simulink model "adsl_sim"  (Simulink 6.0)
settings: Solver=ode45  SolverMode=SingleTasking  StartTime=0.0  StopTime=2  RelTol=1e-3
PreLoadFcn:
  | % variables are initialized through the Model Workspace
model workspace: external: M-Code (data not in the file)
values from neighbouring files (symbols this model uses):
  H = conv2(chCoeff',W)    [eq_computecostfcn.m]    (also in eq_costfcnconverg.m = conv2(eq.chCoeff,W))
undefined symbols (not defined in the file or in its folder): b, rsgenpoly, slcm
libraries: commdigbbndam2 x512, simulink x37, commutil2 x8, commblkcod2 x4, commsequence2 x4, commsink2 x4, commcrc2 x4, commcnvintrlv2 x2, dspxfrm3 x2, dspsrcs4 x2, dspsigattribs x1, dspmtrx3 x1
(part 4 of 5)

== system adsl_sim/DMT Modulator/Modulator Bank 11 ==
  In1 : Inport  LatchInput=off
  Demux1 : Demux  Outputs=b(offset+1:offset+16)
  Matrix Concatenation : simulink/Math Operations/Matrix Concatenation  numInports=16  catMethod=Vertical
  Rectangular QAM Modulator Baseband1 : commdigbbndam2/Rectangular QAM Modulator Baseband  M=2^b(offset+1)  InType=Bit  Enc=Gray  PowType=Average Power  MinDist=2  AvgPow=1  PeakPow=1  Ph=0  numSamp=1
  Rectangular QAM Modulator Baseband10 : commdigbbndam2/Rectangular QAM Modulator Baseband  M=2^b(offset+10)  InType=Bit  Enc=Gray  PowType=Average Power  MinDist=2  AvgPow=1  PeakPow=1  Ph=0  numSamp=1
  Rectangular QAM Modulator Baseband11 : commdigbbndam2/Rectangular QAM Modulator Baseband  M=2^b(offset+11)  InType=Bit  Enc=Gray  PowType=Average Power  MinDist=2  AvgPow=1  PeakPow=1  Ph=0  numSamp=1
  Rectangular QAM Modulator Baseband12 : commdigbbndam2/Rectangular QAM Modulator Baseband  M=2^b(offset+12)  InType=Bit  Enc=Gray  PowType=Average Power  MinDist=2  AvgPow=1  PeakPow=1  Ph=0  numSamp=1
  Rectangular QAM Modulator Baseband13 : commdigbbndam2/Rectangular QAM Modulator Baseband  M=2^b(offset+13)  InType=Bit  Enc=Gray  PowType=Average Power  MinDist=2  AvgPow=1  PeakPow=1  Ph=0  numSamp=1
  Rectangular QAM Modulator Baseband14 : commdigbbndam2/Rectangular QAM Modulator Baseband  M=2^b(offset+14)  InType=Bit  Enc=Gray  PowType=Average Power  MinDist=2  AvgPow=1  PeakPow=1  Ph=0  numSamp=1
  Rectangular QAM Modulator Baseband15 : commdigbbndam2/Rectangular QAM Modulator Baseband  M=2^b(offset+15)  InType=Bit  Enc=Gray  PowType=Average Power  MinDist=2  AvgPow=1  PeakPow=1  Ph=0  numSamp=1
  Rectangular QAM Modulator Baseband16 : commdigbbndam2/Rectangular QAM Modulator Baseband  M=2^b(offset+16)  InType=Bit  Enc=Gray  PowType=Average Power  MinDist=2  AvgPow=1  PeakPow=1  Ph=0  numSamp=1
  Rectangular QAM Modulator Baseband2 : commdigbbndam2/Rectangular QAM Modulator Baseband  M=2^b(offset+2)  InType=Bit  Enc=Gray  PowType=Average Power  MinDist=2  AvgPow=1  PeakPow=1  Ph=0  numSamp=1
  Rectangular QAM Modulator Baseband3 : commdigbbndam2/Rectangular QAM Modulator Baseband  M=2^b(offset+3)  InType=Bit  Enc=Gray  PowType=Average Power  MinDist=2  AvgPow=1  PeakPow=1  Ph=0  numSamp=1
  Rectangular QAM Modulator Baseband4 : commdigbbndam2/Rectangular QAM Modulator Baseband  M=2^b(offset+4)  InType=Bit  Enc=Gray  PowType=Average Power  MinDist=2  AvgPow=1  PeakPow=1  Ph=0  numSamp=1
  Rectangular QAM Modulator Baseband5 : commdigbbndam2/Rectangular QAM Modulator Baseband  M=2^b(offset+5)  InType=Bit  Enc=Gray  PowType=Average Power  MinDist=2  AvgPow=1  PeakPow=1  Ph=0  numSamp=1
  Rectangular QAM Modulator Baseband6 : commdigbbndam2/Rectangular QAM Modulator Baseband  M=2^b(offset+6)  InType=Bit  Enc=Gray  PowType=Average Power  MinDist=2  AvgPow=1  PeakPow=1  Ph=0  numSamp=1
  Rectangular QAM Modulator Baseband7 : commdigbbndam2/Rectangular QAM Modulator Baseband  M=2^b(offset+7)  InType=Bit  Enc=Gray  PowType=Average Power  MinDist=2  AvgPow=1  PeakPow=1  Ph=0  numSamp=1
  Rectangular QAM Modulator Baseband8 : commdigbbndam2/Rectangular QAM Modulator Baseband  M=2^b(offset+8)  InType=Bit  Enc=Gray  PowType=Average Power  MinDist=2  AvgPow=1  PeakPow=1  Ph=0  numSamp=1
  Rectangular QAM Modulator Baseband9 : commdigbbndam2/Rectangular QAM Modulator Baseband  M=2^b(offset+9)  InType=Bit  Enc=Gray  PowType=Average Power  MinDist=2  AvgPow=1  PeakPow=1  Ph=0  numSamp=1
  Out1 : Outport
  wires:
  Rectangular QAM Modulator Baseband16/1 -> Matrix Concatenation/16
  Rectangular QAM Modulator Baseband15/1 -> Matrix Concatenation/15
  Rectangular QAM Modulator Baseband14/1 -> Matrix Concatenation/14
  Rectangular QAM Modulator Baseband13/1 -> Matrix Concatenation/13
  Rectangular QAM Modulator Baseband12/1 -> Matrix Concatenation/12
  Rectangular QAM Modulator Baseband11/1 -> Matrix Concatenation/11
  Rectangular QAM Modulator Baseband10/1 -> Matrix Concatenation/10
  Rectangular QAM Modulator Baseband9/1 -> Matrix Concatenation/9
  Rectangular QAM Modulator Baseband8/1 -> Matrix Concatenation/8
  Rectangular QAM Modulator Baseband7/1 -> Matrix Concatenation/7
  Rectangular QAM Modulator Baseband6/1 -> Matrix Concatenation/6
  Rectangular QAM Modulator Baseband5/1 -> Matrix Concatenation/5
  Rectangular QAM Modulator Baseband4/1 -> Matrix Concatenation/4
  Rectangular QAM Modulator Baseband3/1 -> Matrix Concatenation/3
  Rectangular QAM Modulator Baseband2/1 -> Matrix Concatenation/2
  Demux1/16 -> Rectangular QAM Modulator Baseband16/1
  Demux1/15 -> Rectangular QAM Modulator Baseband15/1
  Demux1/14 -> Rectangular QAM Modulator Baseband14/1
  Demux1/13 -> Rectangular QAM Modulator Baseband13/1
  Demux1/12 -> Rectangular QAM Modulator Baseband12/1
  Demux1/11 -> Rectangular QAM Modulator Baseband11/1
  Demux1/10 -> Rectangular QAM Modulator Baseband10/1
  Demux1/9 -> Rectangular QAM Modulator Baseband9/1
  Demux1/8 -> Rectangular QAM Modulator Baseband8/1
  Demux1/7 -> Rectangular QAM Modulator Baseband7/1
  Demux1/6 -> Rectangular QAM Modulator Baseband6/1
  Demux1/5 -> Rectangular QAM Modulator Baseband5/1
  Demux1/4 -> Rectangular QAM Modulator Baseband4/1
  Demux1/3 -> Rectangular QAM Modulator Baseband3/1
  Matrix Concatenation/1 -> Out1/1
  In1/1 -> Demux1/1
  Demux1/2 -> Rectangular QAM Modulator Baseband2/1
  Demux1/1 -> Rectangular QAM Modulator Baseband1/1
  Rectangular QAM Modulator Baseband1/1 -> Matrix Concatenation/1

== system adsl_sim/DMT Modulator/Modulator Bank 12 ==
  In1 : Inport  LatchInput=off
  Demux1 : Demux  Outputs=b(offset+1:offset+16)
  Matrix Concatenation : simulink/Math Operations/Matrix Concatenation  numInports=16  catMethod=Vertical
  Rectangular QAM Modulator Baseband1 : commdigbbndam2/Rectangular QAM Modulator Baseband  M=2^b(offset+1)  InType=Bit  Enc=Gray  PowType=Average Power  MinDist=2  AvgPow=1  PeakPow=1  Ph=0  numSamp=1
  Rectangular QAM Modulator Baseband10 : commdigbbndam2/Rectangular QAM Modulator Baseband  M=2^b(offset+10)  InType=Bit  Enc=Gray  PowType=Average Power  MinDist=2  AvgPow=1  PeakPow=1  Ph=0  numSamp=1
  Rectangular QAM Modulator Baseband11 : commdigbbndam2/Rectangular QAM Modulator Baseband  M=2^b(offset+11)  InType=Bit  Enc=Gray  PowType=Average Power  MinDist=2  AvgPow=1  PeakPow=1  Ph=0  numSamp=1
  Rectangular QAM Modulator Baseband12 : commdigbbndam2/Rectangular QAM Modulator Baseband  M=2^b(offset+12)  InType=Bit  Enc=Gray  PowType=Average Power  MinDist=2  AvgPow=1  PeakPow=1  Ph=0  numSamp=1
  Rectangular QAM Modulator Baseband13 : commdigbbndam2/Rectangular QAM Modulator Baseband  M=2^b(offset+13)  InType=Bit  Enc=Gray  PowType=Average Power  MinDist=2  AvgPow=1  PeakPow=1  Ph=0  numSamp=1
  Rectangular QAM Modulator Baseband14 : commdigbbndam2/Rectangular QAM Modulator Baseband  M=2^b(offset+14)  InType=Bit  Enc=Gray  PowType=Average Power  MinDist=2  AvgPow=1  PeakPow=1  Ph=0  numSamp=1
  Rectangular QAM Modulator Baseband15 : commdigbbndam2/Rectangular QAM Modulator Baseband  M=2^b(offset+15)  InType=Bit  Enc=Gray  PowType=Average Power  MinDist=2  AvgPow=1  PeakPow=1  Ph=0  numSamp=1
  Rectangular QAM Modulator Baseband16 : commdigbbndam2/Rectangular QAM Modulator Baseband  M=2^b(offset+16)  InType=Bit  Enc=Gray  PowType=Average Power  MinDist=2  AvgPow=1  PeakPow=1  Ph=0  numSamp=1
  Rectangular QAM Modulator Baseband2 : commdigbbndam2/Rectangular QAM Modulator Baseband  M=2^b(offset+2)  InType=Bit  Enc=Gray  PowType=Average Power  MinDist=2  AvgPow=1  PeakPow=1  Ph=0  numSamp=1
  Rectangular QAM Modulator Baseband3 : commdigbbndam2/Rectangular QAM Modulator Baseband  M=2^b(offset+3)  InType=Bit  Enc=Gray  PowType=Average Power  MinDist=2  AvgPow=1  PeakPow=1  Ph=0  numSamp=1
  Rectangular QAM Modulator Baseband4 : commdigbbndam2/Rectangular QAM Modulator Baseband  M=2^b(offset+4)  InType=Bit  Enc=Gray  PowType=Average Power  MinDist=2  AvgPow=1  PeakPow=1  Ph=0  numSamp=1
  Rectangular QAM Modulator Baseband5 : commdigbbndam2/Rectangular QAM Modulator Baseband  M=2^b(offset+5)  InType=Bit  Enc=Gray  PowType=Average Power  MinDist=2  AvgPow=1  PeakPow=1  Ph=0  numSamp=1
  Rectangular QAM Modulator Baseband6 : commdigbbndam2/Rectangular QAM Modulator Baseband  M=2^b(offset+6)  InType=Bit  Enc=Gray  PowType=Average Power  MinDist=2  AvgPow=1  PeakPow=1  Ph=0  numSamp=1
  Rectangular QAM Modulator Baseband7 : commdigbbndam2/Rectangular QAM Modulator Baseband  M=2^b(offset+7)  InType=Bit  Enc=Gray  PowType=Average Power  MinDist=2  AvgPow=1  PeakPow=1  Ph=0  numSamp=1
  Rectangular QAM Modulator Baseband8 : commdigbbndam2/Rectangular QAM Modulator Baseband  M=2^b(offset+8)  InType=Bit  Enc=Gray  PowType=Average Power  MinDist=2  AvgPow=1  PeakPow=1  Ph=0  numSamp=1
  Rectangular QAM Modulator Baseband9 : commdigbbndam2/Rectangular QAM Modulator Baseband  M=2^b(offset+9)  InType=Bit  Enc=Gray  PowType=Average Power  MinDist=2  AvgPow=1  PeakPow=1  Ph=0  numSamp=1
  Out1 : Outport
  wires:
  Rectangular QAM Modulator Baseband1/1 -> Matrix Concatenation/1
  Demux1/1 -> Rectangular QAM Modulator Baseband1/1
  Demux1/2 -> Rectangular QAM Modulator Baseband2/1
  In1/1 -> Demux1/1
  Matrix Concatenation/1 -> Out1/1
  Demux1/3 -> Rectangular QAM Modulator Baseband3/1
  Demux1/4 -> Rectangular QAM Modulator Baseband4/1
  Demux1/5 -> Rectangular QAM Modulator Baseband5/1
  Demux1/6 -> Rectangular QAM Modulator Baseband6/1
  Demux1/7 -> Rectangular QAM Modulator Baseband7/1
  Demux1/8 -> Rectangular QAM Modulator Baseband8/1
  Demux1/9 -> Rectangular QAM Modulator Baseband9/1
  Demux1/10 -> Rectangular QAM Modulator Baseband10/1
  Demux1/11 -> Rectangular QAM Modulator Baseband11/1
  Demux1/12 -> Rectangular QAM Modulator Baseband12/1
  Demux1/13 -> Rectangular QAM Modulator Baseband13/1
  Demux1/14 -> Rectangular QAM Modulator Baseband14/1
  Demux1/15 -> Rectangular QAM Modulator Baseband15/1
  Demux1/16 -> Rectangular QAM Modulator Baseband16/1
  Rectangular QAM Modulator Baseband2/1 -> Matrix Concatenation/2
  Rectangular QAM Modulator Baseband3/1 -> Matrix Concatenation/3
  Rectangular QAM Modulator Baseband4/1 -> Matrix Concatenation/4
  Rectangular QAM Modulator Baseband5/1 -> Matrix Concatenation/5
  Rectangular QAM Modulator Baseband6/1 -> Matrix Concatenation/6
  Rectangular QAM Modulator Baseband7/1 -> Matrix Concatenation/7
  Rectangular QAM Modulator Baseband8/1 -> Matrix Concatenation/8
  Rectangular QAM Modulator Baseband9/1 -> Matrix Concatenation/9
  Rectangular QAM Modulator Baseband10/1 -> Matrix Concatenation/10
  Rectangular QAM Modulator Baseband11/1 -> Matrix Concatenation/11
  Rectangular QAM Modulator Baseband12/1 -> Matrix Concatenation/12
  Rectangular QAM Modulator Baseband13/1 -> Matrix Concatenation/13
  Rectangular QAM Modulator Baseband14/1 -> Matrix Concatenation/14
  Rectangular QAM Modulator Baseband15/1 -> Matrix Concatenation/15
  Rectangular QAM Modulator Baseband16/1 -> Matrix Concatenation/16

== system adsl_sim/DMT Modulator/Modulator Bank 13 ==
  In1 : Inport  LatchInput=off
  Demux1 : Demux  Outputs=b(offset+1:offset+16)
  Matrix Concatenation : simulink/Math Operations/Matrix Concatenation  numInports=16  catMethod=Vertical
  Rectangular QAM Modulator Baseband1 : commdigbbndam2/Rectangular QAM Modulator Baseband  M=2^b(offset+1)  InType=Bit  Enc=Gray  PowType=Average Power  MinDist=2  AvgPow=1  PeakPow=1  Ph=0  numSamp=1
  Rectangular QAM Modulator Baseband10 : commdigbbndam2/Rectangular QAM Modulator Baseband  M=2^b(offset+10)  InType=Bit  Enc=Gray  PowType=Average Power  MinDist=2  AvgPow=1  PeakPow=1  Ph=0  numSamp=1
  Rectangular QAM Modulator Baseband11 : commdigbbndam2/Rectangular QAM Modulator Baseband  M=2^b(offset+11)  InType=Bit  Enc=Gray  PowType=Average Power  MinDist=2  AvgPow=1  PeakPow=1  Ph=0  numSamp=1
  Rectangular QAM Modulator Baseband12 : commdigbbndam2/Rectangular QAM Modulator Baseband  M=2^b(offset+12)  InType=Bit  Enc=Gray  PowType=Average Power  MinDist=2  AvgPow=1  PeakPow=1  Ph=0  numSamp=1
  Rectangular QAM Modulator Baseband13 : commdigbbndam2/Rectangular QAM Modulator Baseband  M=2^b(offset+13)  InType=Bit  Enc=Gray  PowType=Average Power  MinDist=2  AvgPow=1  PeakPow=1  Ph=0  numSamp=1
  Rectangular QAM Modulator Baseband14 : commdigbbndam2/Rectangular QAM Modulator Baseband  M=2^b(offset+14)  InType=Bit  Enc=Gray  PowType=Average Power  MinDist=2  AvgPow=1  PeakPow=1  Ph=0  numSamp=1
  Rectangular QAM Modulator Baseband15 : commdigbbndam2/Rectangular QAM Modulator Baseband  M=2^b(offset+15)  InType=Bit  Enc=Gray  PowType=Average Power  MinDist=2  AvgPow=1  PeakPow=1  Ph=0  numSamp=1
  Rectangular QAM Modulator Baseband16 : commdigbbndam2/Rectangular QAM Modulator Baseband  M=2^b(offset+16)  InType=Bit  Enc=Gray  PowType=Average Power  MinDist=2  AvgPow=1  PeakPow=1  Ph=0  numSamp=1
  Rectangular QAM Modulator Baseband2 : commdigbbndam2/Rectangular QAM Modulator Baseband  M=2^b(offset+2)  InType=Bit  Enc=Gray  PowType=Average Power  MinDist=2  AvgPow=1  PeakPow=1  Ph=0  numSamp=1
  Rectangular QAM Modulator Baseband3 : commdigbbndam2/Rectangular QAM Modulator Baseband  M=2^b(offset+3)  InType=Bit  Enc=Gray  PowType=Average Power  MinDist=2  AvgPow=1  PeakPow=1  Ph=0  numSamp=1
  Rectangular QAM Modulator Baseband4 : commdigbbndam2/Rectangular QAM Modulator Baseband  M=2^b(offset+4)  InType=Bit  Enc=Gray  PowType=Average Power  MinDist=2  AvgPow=1  PeakPow=1  Ph=0  numSamp=1
  Rectangular QAM Modulator Baseband5 : commdigbbndam2/Rectangular QAM Modulator Baseband  M=2^b(offset+5)  InType=Bit  Enc=Gray  PowType=Average Power  MinDist=2  AvgPow=1  PeakPow=1  Ph=0  numSamp=1
  Rectangular QAM Modulator Baseband6 : commdigbbndam2/Rectangular QAM Modulator Baseband  M=2^b(offset+6)  InType=Bit  Enc=Gray  PowType=Average Power  MinDist=2  AvgPow=1  PeakPow=1  Ph=0  numSamp=1
  Rectangular QAM Modulator Baseband7 : commdigbbndam2/Rectangular QAM Modulator Baseband  M=2^b(offset+7)  InType=Bit  Enc=Gray  PowType=Average Power  MinDist=2  AvgPow=1  PeakPow=1  Ph=0  numSamp=1
  Rectangular QAM Modulator Baseband8 : commdigbbndam2/Rectangular QAM Modulator Baseband  M=2^b(offset+8)  InType=Bit  Enc=Gray  PowType=Average Power  MinDist=2  AvgPow=1  PeakPow=1  Ph=0  numSamp=1
  Rectangular QAM Modulator Baseband9 : commdigbbndam2/Rectangular QAM Modulator Baseband  M=2^b(offset+9)  InType=Bit  Enc=Gray  PowType=Average Power  MinDist=2  AvgPow=1  PeakPow=1  Ph=0  numSamp=1
  Out1 : Outport
  wires:
  Rectangular QAM Modulator Baseband16/1 -> Matrix Concatenation/16
  Rectangular QAM Modulator Baseband15/1 -> Matrix Concatenation/15
  Rectangular QAM Modulator Baseband14/1 -> Matrix Concatenation/14
  Rectangular QAM Modulator Baseband13/1 -> Matrix Concatenation/13
  Rectangular QAM Modulator Baseband12/1 -> Matrix Concatenation/12
  Rectangular QAM Modulator Baseband11/1 -> Matrix Concatenation/11
  Rectangular QAM Modulator Baseband10/1 -> Matrix Concatenation/10
  Rectangular QAM Modulator Baseband9/1 -> Matrix Concatenation/9
  Rectangular QAM Modulator Baseband8/1 -> Matrix Concatenation/8
  Rectangular QAM Modulator Baseband7/1 -> Matrix Concatenation/7
  Rectangular QAM Modulator Baseband6/1 -> Matrix Concatenation/6
  Rectangular QAM Modulator Baseband5/1 -> Matrix Concatenation/5
  Rectangular QAM Modulator Baseband4/1 -> Matrix Concatenation/4
  Rectangular QAM Modulator Baseband3/1 -> Matrix Concatenation/3
  Rectangular QAM Modulator Baseband2/1 -> Matrix Concatenation/2
  Demux1/16 -> Rectangular QAM Modulator Baseband16/1
  Demux1/15 -> Rectangular QAM Modulator Baseband15/1
  Demux1/14 -> Rectangular QAM Modulator Baseband14/1
  Demux1/13 -> Rectangular QAM Modulator Baseband13/1
  Demux1/12 -> Rectangular QAM Modulator Baseband12/1
  Demux1/11 -> Rectangular QAM Modulator Baseband11/1
  Demux1/10 -> Rectangular QAM Modulator Baseband10/1
  Demux1/9 -> Rectangular QAM Modulator Baseband9/1
  Demux1/8 -> Rectangular QAM Modulator Baseband8/1
  Demux1/7 -> Rectangular QAM Modulator Baseband7/1
  Demux1/6 -> Rectangular QAM Modulator Baseband6/1
  Demux1/5 -> Rectangular QAM Modulator Baseband5/1
  Demux1/4 -> Rectangular QAM Modulator Baseband4/1
  Demux1/3 -> Rectangular QAM Modulator Baseband3/1
  Matrix Concatenation/1 -> Out1/1
  In1/1 -> Demux1/1
  Demux1/2 -> Rectangular QAM Modulator Baseband2/1
  Demux1/1 -> Rectangular QAM Modulator Baseband1/1
  Rectangular QAM Modulator Baseband1/1 -> Matrix Concatenation/1

== system adsl_sim/DMT Modulator/Modulator Bank 14 ==
  In1 : Inport  LatchInput=off
  Demux1 : Demux  Outputs=b(offset+1:offset+16)
  Matrix Concatenation : simulink/Math Operations/Matrix Concatenation  numInports=16  catMethod=Vertical
  Rectangular QAM Modulator Baseband1 : commdigbbndam2/Rectangular QAM Modulator Baseband  M=2^b(offset+1)  InType=Bit  Enc=Gray  PowType=Average Power  MinDist=2  AvgPow=1  PeakPow=1  Ph=0  numSamp=1
  Rectangular QAM Modulator Baseband10 : commdigbbndam2/Rectangular QAM Modulator Baseband  M=2^b(offset+10)  InType=Bit  Enc=Gray  PowType=Average Power  MinDist=2  AvgPow=1  PeakPow=1  Ph=0  numSamp=1
  Rectangular QAM Modulator Baseband11 : commdigbbndam2/Rectangular QAM Modulator Baseband  M=2^b(offset+11)  InType=Bit  Enc=Gray  PowType=Average Power  MinDist=2  AvgPow=1  PeakPow=1  Ph=0  numSamp=1
  Rectangular QAM Modulator Baseband12 : commdigbbndam2/Rectangular QAM Modulator Baseband  M=2^b(offset+12)  InType=Bit  Enc=Gray  PowType=Average Power  MinDist=2  AvgPow=1  PeakPow=1  Ph=0  numSamp=1
  Rectangular QAM Modulator Baseband13 : commdigbbndam2/Rectangular QAM Modulator Baseband  M=2^b(offset+13)  InType=Bit  Enc=Gray  PowType=Average Power  MinDist=2  AvgPow=1  PeakPow=1  Ph=0  numSamp=1
  Rectangular QAM Modulator Baseband14 : commdigbbndam2/Rectangular QAM Modulator Baseband  M=2^b(offset+14)  InType=Bit  Enc=Gray  PowType=Average Power  MinDist=2  AvgPow=1  PeakPow=1  Ph=0  numSamp=1
  Rectangular QAM Modulator Baseband15 : commdigbbndam2/Rectangular QAM Modulator Baseband  M=2^b(offset+15)  InType=Bit  Enc=Gray  PowType=Average Power  MinDist=2  AvgPow=1  PeakPow=1  Ph=0  numSamp=1
  Rectangular QAM Modulator Baseband16 : commdigbbndam2/Rectangular QAM Modulator Baseband  M=2^b(offset+16)  InType=Bit  Enc=Gray  PowType=Average Power  MinDist=2  AvgPow=1  PeakPow=1  Ph=0  numSamp=1
  Rectangular QAM Modulator Baseband2 : commdigbbndam2/Rectangular QAM Modulator Baseband  M=2^b(offset+2)  InType=Bit  Enc=Gray  PowType=Average Power  MinDist=2  AvgPow=1  PeakPow=1  Ph=0  numSamp=1
  Rectangular QAM Modulator Baseband3 : commdigbbndam2/Rectangular QAM Modulator Baseband  M=2^b(offset+3)  InType=Bit  Enc=Gray  PowType=Average Power  MinDist=2  AvgPow=1  PeakPow=1  Ph=0  numSamp=1
  Rectangular QAM Modulator Baseband4 : commdigbbndam2/Rectangular QAM Modulator Baseband  M=2^b(offset+4)  InType=Bit  Enc=Gray  PowType=Average Power  MinDist=2  AvgPow=1  PeakPow=1  Ph=0  numSamp=1
  Rectangular QAM Modulator Baseband5 : commdigbbndam2/Rectangular QAM Modulator Baseband  M=2^b(offset+5)  InType=Bit  Enc=Gray  PowType=Average Power  MinDist=2  AvgPow=1  PeakPow=1  Ph=0  numSamp=1
  Rectangular QAM Modulator Baseband6 : commdigbbndam2/Rectangular QAM Modulator Baseband  M=2^b(offset+6)  InType=Bit  Enc=Gray  PowType=Average Power  MinDist=2  AvgPow=1  PeakPow=1  Ph=0  numSamp=1
  Rectangular QAM Modulator Baseband7 : commdigbbndam2/Rectangular QAM Modulator Baseband  M=2^b(offset+7)  InType=Bit  Enc=Gray  PowType=Average Power  MinDist=2  AvgPow=1  PeakPow=1  Ph=0  numSamp=1
  Rectangular QAM Modulator Baseband8 : commdigbbndam2/Rectangular QAM Modulator Baseband  M=2^b(offset+8)  InType=Bit  Enc=Gray  PowType=Average Power  MinDist=2  AvgPow=1  PeakPow=1  Ph=0  numSamp=1
  Rectangular QAM Modulator Baseband9 : commdigbbndam2/Rectangular QAM Modulator Baseband  M=2^b(offset+9)  InType=Bit  Enc=Gray  PowType=Average Power  MinDist=2  AvgPow=1  PeakPow=1  Ph=0  numSamp=1
  Out1 : Outport
  wires:
  Rectangular QAM Modulator Baseband1/1 -> Matrix Concatenation/1
  Demux1/1 -> Rectangular QAM Modulator Baseband1/1
  Demux1/2 -> Rectangular QAM Modulator Baseband2/1
  In1/1 -> Demux1/1
  Matrix Concatenation/1 -> Out1/1
  Demux1/3 -> Rectangular QAM Modulator Baseband3/1
  Demux1/4 -> Rectangular QAM Modulator Baseband4/1
  Demux1/5 -> Rectangular QAM Modulator Baseband5/1
  Demux1/6 -> Rectangular QAM Modulator Baseband6/1
  Demux1/7 -> Rectangular QAM Modulator Baseband7/1
  Demux1/8 -> Rectangular QAM Modulator Baseband8/1
  Demux1/9 -> Rectangular QAM Modulator Baseband9/1
  Demux1/10 -> Rectangular QAM Modulator Baseband10/1
  Demux1/11 -> Rectangular QAM Modulator Baseband11/1
  Demux1/12 -> Rectangular QAM Modulator Baseband12/1
  Demux1/13 -> Rectangular QAM Modulator Baseband13/1
  Demux1/14 -> Rectangular QAM Modulator Baseband14/1
  Demux1/15 -> Rectangular QAM Modulator Baseband15/1
  Demux1/16 -> Rectangular QAM Modulator Baseband16/1
  Rectangular QAM Modulator Baseband2/1 -> Matrix Concatenation/2
  Rectangular QAM Modulator Baseband3/1 -> Matrix Concatenation/3
  Rectangular QAM Modulator Baseband4/1 -> Matrix Concatenation/4
  Rectangular QAM Modulator Baseband5/1 -> Matrix Concatenation/5
  Rectangular QAM Modulator Baseband6/1 -> Matrix Concatenation/6
  Rectangular QAM Modulator Baseband7/1 -> Matrix Concatenation/7
  Rectangular QAM Modulator Baseband8/1 -> Matrix Concatenation/8
  Rectangular QAM Modulator Baseband9/1 -> Matrix Concatenation/9
  Rectangular QAM Modulator Baseband10/1 -> Matrix Concatenation/10
  Rectangular QAM Modulator Baseband11/1 -> Matrix Concatenation/11
  Rectangular QAM Modulator Baseband12/1 -> Matrix Concatenation/12
  Rectangular QAM Modulator Baseband13/1 -> Matrix Concatenation/13
  Rectangular QAM Modulator Baseband14/1 -> Matrix Concatenation/14
  Rectangular QAM Modulator Baseband15/1 -> Matrix Concatenation/15
  Rectangular QAM Modulator Baseband16/1 -> Matrix Concatenation/16

== system adsl_sim/DMT Modulator/Modulator Bank 15 ==
  In1 : Inport  LatchInput=off
  Demux1 : Demux  Outputs=b(offset+1:offset+16)
  Matrix Concatenation : simulink/Math Operations/Matrix Concatenation  numInports=16  catMethod=Vertical
  Rectangular QAM Modulator Baseband1 : commdigbbndam2/Rectangular QAM Modulator Baseband  M=2^b(offset+1)  InType=Bit  Enc=Gray  PowType=Average Power  MinDist=2  AvgPow=1  PeakPow=1  Ph=0  numSamp=1
  Rectangular QAM Modulator Baseband10 : commdigbbndam2/Rectangular QAM Modulator Baseband  M=2^b(offset+10)  InType=Bit  Enc=Gray  PowType=Average Power  MinDist=2  AvgPow=1  PeakPow=1  Ph=0  numSamp=1
  Rectangular QAM Modulator Baseband11 : commdigbbndam2/Rectangular QAM Modulator Baseband  M=2^b(offset+11)  InType=Bit  Enc=Gray  PowType=Average Power  MinDist=2  AvgPow=1  PeakPow=1  Ph=0  numSamp=1
  Rectangular QAM Modulator Baseband12 : commdigbbndam2/Rectangular QAM Modulator Baseband  M=2^b(offset+12)  InType=Bit  Enc=Gray  PowType=Average Power  MinDist=2  AvgPow=1  PeakPow=1  Ph=0  numSamp=1
  Rectangular QAM Modulator Baseband13 : commdigbbndam2/Rectangular QAM Modulator Baseband  M=2^b(offset+13)  InType=Bit  Enc=Gray  PowType=Average Power  MinDist=2  AvgPow=1  PeakPow=1  Ph=0  numSamp=1
  Rectangular QAM Modulator Baseband14 : commdigbbndam2/Rectangular QAM Modulator Baseband  M=2^b(offset+14)  InType=Bit  Enc=Gray  PowType=Average Power  MinDist=2  AvgPow=1  PeakPow=1  Ph=0  numSamp=1
  Rectangular QAM Modulator Baseband15 : commdigbbndam2/Rectangular QAM Modulator Baseband  M=2^b(offset+15)  InType=Bit  Enc=Gray  PowType=Average Power  MinDist=2  AvgPow=1  PeakPow=1  Ph=0  numSamp=1
  Rectangular QAM Modulator Baseband16 : commdigbbndam2/Rectangular QAM Modulator Baseband  M=2^b(offset+16)  InType=Bit  Enc=Gray  PowType=Average Power  MinDist=2  AvgPow=1  PeakPow=1  Ph=0  numSamp=1
  Rectangular QAM Modulator Baseband2 : commdigbbndam2/Rectangular QAM Modulator Baseband  M=2^b(offset+2)  InType=Bit  Enc=Gray  PowType=Average Power  MinDist=2  AvgPow=1  PeakPow=1  Ph=0  numSamp=1
  Rectangular QAM Modulator Baseband3 : commdigbbndam2/Rectangular QAM Modulator Baseband  M=2^b(offset+3)  InType=Bit  Enc=Gray  PowType=Average Power  MinDist=2  AvgPow=1  PeakPow=1  Ph=0  numSamp=1
  Rectangular QAM Modulator Baseband4 : commdigbbndam2/Rectangular QAM Modulator Baseband  M=2^b(offset+4)  InType=Bit  Enc=Gray  PowType=Average Power  MinDist=2  AvgPow=1  PeakPow=1  Ph=0  numSamp=1
  Rectangular QAM Modulator Baseband5 : commdigbbndam2/Rectangular QAM Modulator Baseband  M=2^b(offset+5)  InType=Bit  Enc=Gray  PowType=Average Power  MinDist=2  AvgPow=1  PeakPow=1  Ph=0  numSamp=1
  Rectangular QAM Modulator Baseband6 : commdigbbndam2/Rectangular QAM Modulator Baseband  M=2^b(offset+6)  InType=Bit  Enc=Gray  PowType=Average Power  MinDist=2  AvgPow=1  PeakPow=1  Ph=0  numSamp=1
  Rectangular QAM Modulator Baseband7 : commdigbbndam2/Rectangular QAM Modulator Baseband  M=2^b(offset+7)  InType=Bit  Enc=Gray  PowType=Average Power  MinDist=2  AvgPow=1  PeakPow=1  Ph=0  numSamp=1
  Rectangular QAM Modulator Baseband8 : commdigbbndam2/Rectangular QAM Modulator Baseband  M=2^b(offset+8)  InType=Bit  Enc=Gray  PowType=Average Power  MinDist=2  AvgPow=1  PeakPow=1  Ph=0  numSamp=1
  Rectangular QAM Modulator Baseband9 : commdigbbndam2/Rectangular QAM Modulator Baseband  M=2^b(offset+9)  InType=Bit  Enc=Gray  PowType=Average Power  MinDist=2  AvgPow=1  PeakPow=1  Ph=0  numSamp=1
  Out1 : Outport
  wires:
  Rectangular QAM Modulator Baseband16/1 -> Matrix Concatenation/16
  Rectangular QAM Modulator Baseband15/1 -> Matrix Concatenation/15
  Rectangular QAM Modulator Baseband14/1 -> Matrix Concatenation/14
  Rectangular QAM Modulator Baseband13/1 -> Matrix Concatenation/13
  Rectangular QAM Modulator Baseband12/1 -> Matrix Concatenation/12
  Rectangular QAM Modulator Baseband11/1 -> Matrix Concatenation/11
  Rectangular QAM Modulator Baseband10/1 -> Matrix Concatenation/10
  Rectangular QAM Modulator Baseband9/1 -> Matrix Concatenation/9
  Rectangular QAM Modulator Baseband8/1 -> Matrix Concatenation/8
  Rectangular QAM Modulator Baseband7/1 -> Matrix Concatenation/7
  Rectangular QAM Modulator Baseband6/1 -> Matrix Concatenation/6
  Rectangular QAM Modulator Baseband5/1 -> Matrix Concatenation/5
  Rectangular QAM Modulator Baseband4/1 -> Matrix Concatenation/4
  Rectangular QAM Modulator Baseband3/1 -> Matrix Concatenation/3
  Rectangular QAM Modulator Baseband2/1 -> Matrix Concatenation/2
  Demux1/16 -> Rectangular QAM Modulator Baseband16/1
  Demux1/15 -> Rectangular QAM Modulator Baseband15/1
  Demux1/14 -> Rectangular QAM Modulator Baseband14/1
  Demux1/13 -> Rectangular QAM Modulator Baseband13/1
  Demux1/12 -> Rectangular QAM Modulator Baseband12/1
  Demux1/11 -> Rectangular QAM Modulator Baseband11/1
  Demux1/10 -> Rectangular QAM Modulator Baseband10/1
  Demux1/9 -> Rectangular QAM Modulator Baseband9/1
  Demux1/8 -> Rectangular QAM Modulator Baseband8/1
  Demux1/7 -> Rectangular QAM Modulator Baseband7/1
  Demux1/6 -> Rectangular QAM Modulator Baseband6/1
  Demux1/5 -> Rectangular QAM Modulator Baseband5/1
  Demux1/4 -> Rectangular QAM Modulator Baseband4/1
  Demux1/3 -> Rectangular QAM Modulator Baseband3/1
  Matrix Concatenation/1 -> Out1/1
  In1/1 -> Demux1/1
  Demux1/2 -> Rectangular QAM Modulator Baseband2/1
  Demux1/1 -> Rectangular QAM Modulator Baseband1/1
  Rectangular QAM Modulator Baseband1/1 -> Matrix Concatenation/1

== system adsl_sim/DMT Modulator/Modulator Bank 16 ==
  In1 : Inport  LatchInput=off
  Demux1 : Demux  Outputs=b(offset+1:offset+16)
  Matrix Concatenation : simulink/Math Operations/Matrix Concatenation  numInports=16  catMethod=Vertical
  Rectangular QAM Modulator Baseband1 : commdigbbndam2/Rectangular QAM Modulator Baseband  M=2^b(offset+1)  InType=Bit  Enc=Gray  PowType=Average Power  MinDist=2  AvgPow=1  PeakPow=1  Ph=0  numSamp=1
  Rectangular QAM Modulator Baseband10 : commdigbbndam2/Rectangular QAM Modulator Baseband  M=2^b(offset+10)  InType=Bit  Enc=Gray  PowType=Average Power  MinDist=2  AvgPow=1  PeakPow=1  Ph=0  numSamp=1
  Rectangular QAM Modulator Baseband11 : commdigbbndam2/Rectangular QAM Modulator Baseband  M=2^b(offset+11)  InType=Bit  Enc=Gray  PowType=Average Power  MinDist=2  AvgPow=1  PeakPow=1  Ph=0  numSamp=1
  Rectangular QAM Modulator Baseband12 : commdigbbndam2/Rectangular QAM Modulator Baseband  M=2^b(offset+12)  InType=Bit  Enc=Gray  PowType=Average Power  MinDist=2  AvgPow=1  PeakPow=1  Ph=0  numSamp=1
  Rectangular QAM Modulator Baseband13 : commdigbbndam2/Rectangular QAM Modulator Baseband  M=2^b(offset+13)  InType=Bit  Enc=Gray  PowType=Average Power  MinDist=2  AvgPow=1  PeakPow=1  Ph=0  numSamp=1
  Rectangular QAM Modulator Baseband14 : commdigbbndam2/Rectangular QAM Modulator Baseband  M=2^b(offset+14)  InType=Bit  Enc=Gray  PowType=Average Power  MinDist=2  AvgPow=1  PeakPow=1  Ph=0  numSamp=1
  Rectangular QAM Modulator Baseband15 : commdigbbndam2/Rectangular QAM Modulator Baseband  M=2^b(offset+15)  InType=Bit  Enc=Gray  PowType=Average Power  MinDist=2  AvgPow=1  PeakPow=1  Ph=0  numSamp=1
  Rectangular QAM Modulator Baseband16 : commdigbbndam2/Rectangular QAM Modulator Baseband  M=2^b(offset+16)  InType=Bit  Enc=Gray  PowType=Average Power  MinDist=2  AvgPow=1  PeakPow=1  Ph=0  numSamp=1
  Rectangular QAM Modulator Baseband2 : commdigbbndam2/Rectangular QAM Modulator Baseband  M=2^b(offset+2)  InType=Bit  Enc=Gray  PowType=Average Power  MinDist=2  AvgPow=1  PeakPow=1  Ph=0  numSamp=1
  Rectangular QAM Modulator Baseband3 : commdigbbndam2/Rectangular QAM Modulator Baseband  M=2^b(offset+3)  InType=Bit  Enc=Gray  PowType=Average Power  MinDist=2  AvgPow=1  PeakPow=1  Ph=0  numSamp=1
  Rectangular QAM Modulator Baseband4 : commdigbbndam2/Rectangular QAM Modulator Baseband  M=2^b(offset+4)  InType=Bit  Enc=Gray  PowType=Average Power  MinDist=2  AvgPow=1  PeakPow=1  Ph=0  numSamp=1
  Rectangular QAM Modulator Baseband5 : commdigbbndam2/Rectangular QAM Modulator Baseband  M=2^b(offset+5)  InType=Bit  Enc=Gray  PowType=Average Power  MinDist=2  AvgPow=1  PeakPow=1  Ph=0  numSamp=1
  Rectangular QAM Modulator Baseband6 : commdigbbndam2/Rectangular QAM Modulator Baseband  M=2^b(offset+6)  InType=Bit  Enc=Gray  PowType=Average Power  MinDist=2  AvgPow=1  PeakPow=1  Ph=0  numSamp=1
  Rectangular QAM Modulator Baseband7 : commdigbbndam2/Rectangular QAM Modulator Baseband  M=2^b(offset+7)  InType=Bit  Enc=Gray  PowType=Average Power  MinDist=2  AvgPow=1  PeakPow=1  Ph=0  numSamp=1
  Rectangular QAM Modulator Baseband8 : commdigbbndam2/Rectangular QAM Modulator Baseband  M=2^b(offset+8)  InType=Bit  Enc=Gray  PowType=Average Power  MinDist=2  AvgPow=1  PeakPow=1  Ph=0  numSamp=1
  Rectangular QAM Modulator Baseband9 : commdigbbndam2/Rectangular QAM Modulator Baseband  M=2^b(offset+9)  InType=Bit  Enc=Gray  PowType=Average Power  MinDist=2  AvgPow=1  PeakPow=1  Ph=0  numSamp=1
  Out1 : Outport
  wires:
  Rectangular QAM Modulator Baseband1/1 -> Matrix Concatenation/1
  Demux1/1 -> Rectangular QAM Modulator Baseband1/1
  Demux1/2 -> Rectangular QAM Modulator Baseband2/1
  In1/1 -> Demux1/1
  Matrix Concatenation/1 -> Out1/1
  Demux1/3 -> Rectangular QAM Modulator Baseband3/1
  Demux1/4 -> Rectangular QAM Modulator Baseband4/1
  Demux1/5 -> Rectangular QAM Modulator Baseband5/1
  Demux1/6 -> Rectangular QAM Modulator Baseband6/1
  Demux1/7 -> Rectangular QAM Modulator Baseband7/1
  Demux1/8 -> Rectangular QAM Modulator Baseband8/1
  Demux1/9 -> Rectangular QAM Modulator Baseband9/1
  Demux1/10 -> Rectangular QAM Modulator Baseband10/1
  Demux1/11 -> Rectangular QAM Modulator Baseband11/1
  Demux1/12 -> Rectangular QAM Modulator Baseband12/1
  Demux1/13 -> Rectangular QAM Modulator Baseband13/1
  Demux1/14 -> Rectangular QAM Modulator Baseband14/1
  Demux1/15 -> Rectangular QAM Modulator Baseband15/1
  Demux1/16 -> Rectangular QAM Modulator Baseband16/1
  Rectangular QAM Modulator Baseband2/1 -> Matrix Concatenation/2
  Rectangular QAM Modulator Baseband3/1 -> Matrix Concatenation/3
  Rectangular QAM Modulator Baseband4/1 -> Matrix Concatenation/4
  Rectangular QAM Modulator Baseband5/1 -> Matrix Concatenation/5
  Rectangular QAM Modulator Baseband6/1 -> Matrix Concatenation/6
  Rectangular QAM Modulator Baseband7/1 -> Matrix Concatenation/7
  Rectangular QAM Modulator Baseband8/1 -> Matrix Concatenation/8
  Rectangular QAM Modulator Baseband9/1 -> Matrix Concatenation/9
  Rectangular QAM Modulator Baseband10/1 -> Matrix Concatenation/10
  Rectangular QAM Modulator Baseband11/1 -> Matrix Concatenation/11
  Rectangular QAM Modulator Baseband12/1 -> Matrix Concatenation/12
  Rectangular QAM Modulator Baseband13/1 -> Matrix Concatenation/13
  Rectangular QAM Modulator Baseband14/1 -> Matrix Concatenation/14
  Rectangular QAM Modulator Baseband15/1 -> Matrix Concatenation/15
  Rectangular QAM Modulator Baseband16/1 -> Matrix Concatenation/16

== system adsl_sim/DMT Modulator/Modulator Bank 2 ==
  In1 : Inport  LatchInput=off
  Demux1 : Demux  Outputs=b(offset+1:offset+16)
  Matrix Concatenation : simulink/Math Operations/Matrix Concatenation  numInports=16  catMethod=Vertical
  Rectangular QAM Modulator Baseband1 : commdigbbndam2/Rectangular QAM Modulator Baseband  M=2^b(offset+1)  InType=Bit  Enc=Gray  PowType=Average Power  MinDist=2  AvgPow=1  PeakPow=1  Ph=0  numSamp=1
  Rectangular QAM Modulator Baseband10 : commdigbbndam2/Rectangular QAM Modulator Baseband  M=2^b(offset+10)  InType=Bit  Enc=Gray  PowType=Average Power  MinDist=2  AvgPow=1  PeakPow=1  Ph=0  numSamp=1
  Rectangular QAM Modulator Baseband11 : commdigbbndam2/Rectangular QAM Modulator Baseband  M=2^b(offset+11)  InType=Bit  Enc=Gray  PowType=Average Power  MinDist=2  AvgPow=1  PeakPow=1  Ph=0  numSamp=1
  Rectangular QAM Modulator Baseband12 : commdigbbndam2/Rectangular QAM Modulator Baseband  M=2^b(offset+12)  InType=Bit  Enc=Gray  PowType=Average Power  MinDist=2  AvgPow=1  PeakPow=1  Ph=0  numSamp=1
  Rectangular QAM Modulator Baseband13 : commdigbbndam2/Rectangular QAM Modulator Baseband  M=2^b(offset+13)  InType=Bit  Enc=Gray  PowType=Average Power  MinDist=2  AvgPow=1  PeakPow=1  Ph=0  numSamp=1
  Rectangular QAM Modulator Baseband14 : commdigbbndam2/Rectangular QAM Modulator Baseband  M=2^b(offset+14)  InType=Bit  Enc=Gray  PowType=Average Power  MinDist=2  AvgPow=1  PeakPow=1  Ph=0  numSamp=1
  Rectangular QAM Modulator Baseband15 : commdigbbndam2/Rectangular QAM Modulator Baseband  M=2^b(offset+15)  InType=Bit  Enc=Gray  PowType=Average Power  MinDist=2  AvgPow=1  PeakPow=1  Ph=0  numSamp=1
  Rectangular QAM Modulator Baseband16 : commdigbbndam2/Rectangular QAM Modulator Baseband  M=2^b(offset+16)  InType=Bit  Enc=Gray  PowType=Average Power  MinDist=2  AvgPow=1  PeakPow=1  Ph=0  numSamp=1
  Rectangular QAM Modulator Baseband2 : commdigbbndam2/Rectangular QAM Modulator Baseband  M=2^b(offset+2)  InType=Bit  Enc=Gray  PowType=Average Power  MinDist=2  AvgPow=1  PeakPow=1  Ph=0  numSamp=1
  Rectangular QAM Modulator Baseband3 : commdigbbndam2/Rectangular QAM Modulator Baseband  M=2^b(offset+3)  InType=Bit  Enc=Gray  PowType=Average Power  MinDist=2  AvgPow=1  PeakPow=1  Ph=0  numSamp=1
  Rectangular QAM Modulator Baseband4 : commdigbbndam2/Rectangular QAM Modulator Baseband  M=2^b(offset+4)  InType=Bit  Enc=Gray  PowType=Average Power  MinDist=2  AvgPow=1  PeakPow=1  Ph=0  numSamp=1
  Rectangular QAM Modulator Baseband5 : commdigbbndam2/Rectangular QAM Modulator Baseband  M=2^b(offset+5)  InType=Bit  Enc=Gray  PowType=Average Power  MinDist=2  AvgPow=1  PeakPow=1  Ph=0  numSamp=1
  Rectangular QAM Modulator Baseband6 : commdigbbndam2/Rectangular QAM Modulator Baseband  M=2^b(offset+6)  InType=Bit  Enc=Gray  PowType=Average Power  MinDist=2  AvgPow=1  PeakPow=1  Ph=0  numSamp=1
  Rectangular QAM Modulator Baseband7 : commdigbbndam2/Rectangular QAM Modulator Baseband  M=2^b(offset+7)  InType=Bit  Enc=Gray  PowType=Average Power  MinDist=2  AvgPow=1  PeakPow=1  Ph=0  numSamp=1
  Rectangular QAM Modulator Baseband8 : commdigbbndam2/Rectangular QAM Modulator Baseband  M=2^b(offset+8)  InType=Bit  Enc=Gray  PowType=Average Power  MinDist=2  AvgPow=1  PeakPow=1  Ph=0  numSamp=1
  Rectangular QAM Modulator Baseband9 : commdigbbndam2/Rectangular QAM Modulator Baseband  M=2^b(offset+9)  InType=Bit  Enc=Gray  PowType=Average Power  MinDist=2  AvgPow=1  PeakPow=1  Ph=0  numSamp=1
  Out1 : Outport
  wires:
  Rectangular QAM Modulator Baseband16/1 -> Matrix Concatenation/16
  Rectangular QAM Modulator Baseband15/1 -> Matrix Concatenation/15
  Rectangular QAM Modulator Baseband14/1 -> Matrix Concatenation/14
  Rectangular QAM Modulator Baseband13/1 -> Matrix Concatenation/13
  Rectangular QAM Modulator Baseband12/1 -> Matrix Concatenation/12
  Rectangular QAM Modulator Baseband11/1 -> Matrix Concatenation/11
  Rectangular QAM Modulator Baseband10/1 -> Matrix Concatenation/10
  Rectangular QAM Modulator Baseband9/1 -> Matrix Concatenation/9
  Rectangular QAM Modulator Baseband8/1 -> Matrix Concatenation/8
  Rectangular QAM Modulator Baseband7/1 -> Matrix Concatenation/7
  Rectangular QAM Modulator Baseband6/1 -> Matrix Concatenation/6
  Rectangular QAM Modulator Baseband5/1 -> Matrix Concatenation/5
  Rectangular QAM Modulator Baseband4/1 -> Matrix Concatenation/4
  Rectangular QAM Modulator Baseband3/1 -> Matrix Concatenation/3
  Rectangular QAM Modulator Baseband2/1 -> Matrix Concatenation/2
  Demux1/16 -> Rectangular QAM Modulator Baseband16/1
  Demux1/15 -> Rectangular QAM Modulator Baseband15/1
  Demux1/14 -> Rectangular QAM Modulator Baseband14/1
  Demux1/13 -> Rectangular QAM Modulator Baseband13/1
  Demux1/12 -> Rectangular QAM Modulator Baseband12/1
  Demux1/11 -> Rectangular QAM Modulator Baseband11/1
  Demux1/10 -> Rectangular QAM Modulator Baseband10/1
  Demux1/9 -> Rectangular QAM Modulator Baseband9/1
  Demux1/8 -> Rectangular QAM Modulator Baseband8/1
  Demux1/7 -> Rectangular QAM Modulator Baseband7/1
  Demux1/6 -> Rectangular QAM Modulator Baseband6/1
  Demux1/5 -> Rectangular QAM Modulator Baseband5/1
  Demux1/4 -> Rectangular QAM Modulator Baseband4/1
  Demux1/3 -> Rectangular QAM Modulator Baseband3/1
  Matrix Concatenation/1 -> Out1/1
  In1/1 -> Demux1/1
  Demux1/2 -> Rectangular QAM Modulator Baseband2/1
  Demux1/1 -> Rectangular QAM Modulator Baseband1/1
  Rectangular QAM Modulator Baseband1/1 -> Matrix Concatenation/1

== system adsl_sim/DMT Modulator/Modulator Bank 3 ==
  In1 : Inport  LatchInput=off
  Demux1 : Demux  Outputs=b(offset+1:offset+16)
  Matrix Concatenation : simulink/Math Operations/Matrix Concatenation  numInports=16  catMethod=Vertical
  Rectangular QAM Modulator Baseband1 : commdigbbndam2/Rectangular QAM Modulator Baseband  M=2^b(offset+1)  InType=Bit  Enc=Gray  PowType=Average Power  MinDist=2  AvgPow=1  PeakPow=1  Ph=0  numSamp=1
  Rectangular QAM Modulator Baseband10 : commdigbbndam2/Rectangular QAM Modulator Baseband  M=2^b(offset+10)  InType=Bit  Enc=Gray  PowType=Average Power  MinDist=2  AvgPow=1  PeakPow=1  Ph=0  numSamp=1
  Rectangular QAM Modulator Baseband11 : commdigbbndam2/Rectangular QAM Modulator Baseband  M=2^b(offset+11)  InType=Bit  Enc=Gray  PowType=Average Power  MinDist=2  AvgPow=1  PeakPow=1  Ph=0  numSamp=1
  Rectangular QAM Modulator Baseband12 : commdigbbndam2/Rectangular QAM Modulator Baseband  M=2^b(offset+12)  InType=Bit  Enc=Gray  PowType=Average Power  MinDist=2  AvgPow=1  PeakPow=1  Ph=0  numSamp=1
  Rectangular QAM Modulator Baseband13 : commdigbbndam2/Rectangular QAM Modulator Baseband  M=2^b(offset+13)  InType=Bit  Enc=Gray  PowType=Average Power  MinDist=2  AvgPow=1  PeakPow=1  Ph=0  numSamp=1
  Rectangular QAM Modulator Baseband14 : commdigbbndam2/Rectangular QAM Modulator Baseband  M=2^b(offset+14)  InType=Bit  Enc=Gray  PowType=Average Power  MinDist=2  AvgPow=1  PeakPow=1  Ph=0  numSamp=1
  Rectangular QAM Modulator Baseband15 : commdigbbndam2/Rectangular QAM Modulator Baseband  M=2^b(offset+15)  InType=Bit  Enc=Gray  PowType=Average Power  MinDist=2  AvgPow=1  PeakPow=1  Ph=0  numSamp=1
  Rectangular QAM Modulator Baseband16 : commdigbbndam2/Rectangular QAM Modulator Baseband  M=2^b(offset+16)  InType=Bit  Enc=Gray  PowType=Average Power  MinDist=2  AvgPow=1  PeakPow=1  Ph=0  numSamp=1
  Rectangular QAM Modulator Baseband2 : commdigbbndam2/Rectangular QAM Modulator Baseband  M=2^b(offset+2)  InType=Bit  Enc=Gray  PowType=Average Power  MinDist=2  AvgPow=1  PeakPow=1  Ph=0  numSamp=1
  Rectangular QAM Modulator Baseband3 : commdigbbndam2/Rectangular QAM Modulator Baseband  M=2^b(offset+3)  InType=Bit  Enc=Gray  PowType=Average Power  MinDist=2  AvgPow=1  PeakPow=1  Ph=0  numSamp=1
  Rectangular QAM Modulator Baseband4 : commdigbbndam2/Rectangular QAM Modulator Baseband  M=2^b(offset+4)  InType=Bit  Enc=Gray  PowType=Average Power  MinDist=2  AvgPow=1  PeakPow=1  Ph=0  numSamp=1
  Rectangular QAM Modulator Baseband5 : commdigbbndam2/Rectangular QAM Modulator Baseband  M=2^b(offset+5)  InType=Bit  Enc=Gray  PowType=Average Power  MinDist=2  AvgPow=1  PeakPow=1  Ph=0  numSamp=1
  Rectangular QAM Modulator Baseband6 : commdigbbndam2/Rectangular QAM Modulator Baseband  M=2^b(offset+6)  InType=Bit  Enc=Gray  PowType=Average Power  MinDist=2  AvgPow=1  PeakPow=1  Ph=0  numSamp=1
  Rectangular QAM Modulator Baseband7 : commdigbbndam2/Rectangular QAM Modulator Baseband  M=2^b(offset+7)  InType=Bit  Enc=Gray  PowType=Average Power  MinDist=2  AvgPow=1  PeakPow=1  Ph=0  numSamp=1
  Rectangular QAM Modulator Baseband8 : commdigbbndam2/Rectangular QAM Modulator Baseband  M=2^b(offset+8)  InType=Bit  Enc=Gray  PowType=Average Power  MinDist=2  AvgPow=1  PeakPow=1  Ph=0  numSamp=1
  Rectangular QAM Modulator Baseband9 : commdigbbndam2/Rectangular QAM Modulator Baseband  M=2^b(offset+9)  InType=Bit  Enc=Gray  PowType=Average Power  MinDist=2  AvgPow=1  PeakPow=1  Ph=0  numSamp=1
  Out1 : Outport
  wires:
  Rectangular QAM Modulator Baseband1/1 -> Matrix Concatenation/1
  Demux1/1 -> Rectangular QAM Modulator Baseband1/1
  Demux1/2 -> Rectangular QAM Modulator Baseband2/1
  In1/1 -> Demux1/1
  Matrix Concatenation/1 -> Out1/1
  Demux1/3 -> Rectangular QAM Modulator Baseband3/1
  Demux1/4 -> Rectangular QAM Modulator Baseband4/1
  Demux1/5 -> Rectangular QAM Modulator Baseband5/1
  Demux1/6 -> Rectangular QAM Modulator Baseband6/1
  Demux1/7 -> Rectangular QAM Modulator Baseband7/1
  Demux1/8 -> Rectangular QAM Modulator Baseband8/1
  Demux1/9 -> Rectangular QAM Modulator Baseband9/1
  Demux1/10 -> Rectangular QAM Modulator Baseband10/1
  Demux1/11 -> Rectangular QAM Modulator Baseband11/1
  Demux1/12 -> Rectangular QAM Modulator Baseband12/1
  Demux1/13 -> Rectangular QAM Modulator Baseband13/1
  Demux1/14 -> Rectangular QAM Modulator Baseband14/1
  Demux1/15 -> Rectangular QAM Modulator Baseband15/1
  Demux1/16 -> Rectangular QAM Modulator Baseband16/1
  Rectangular QAM Modulator Baseband2/1 -> Matrix Concatenation/2
  Rectangular QAM Modulator Baseband3/1 -> Matrix Concatenation/3
  Rectangular QAM Modulator Baseband4/1 -> Matrix Concatenation/4
  Rectangular QAM Modulator Baseband5/1 -> Matrix Concatenation/5
  Rectangular QAM Modulator Baseband6/1 -> Matrix Concatenation/6
  Rectangular QAM Modulator Baseband7/1 -> Matrix Concatenation/7
  Rectangular QAM Modulator Baseband8/1 -> Matrix Concatenation/8
  Rectangular QAM Modulator Baseband9/1 -> Matrix Concatenation/9
  Rectangular QAM Modulator Baseband10/1 -> Matrix Concatenation/10
  Rectangular QAM Modulator Baseband11/1 -> Matrix Concatenation/11
  Rectangular QAM Modulator Baseband12/1 -> Matrix Concatenation/12
  Rectangular QAM Modulator Baseband13/1 -> Matrix Concatenation/13
  Rectangular QAM Modulator Baseband14/1 -> Matrix Concatenation/14
  Rectangular QAM Modulator Baseband15/1 -> Matrix Concatenation/15
  Rectangular QAM Modulator Baseband16/1 -> Matrix Concatenation/16

== system adsl_sim/DMT Modulator/Modulator Bank 4 ==
  In1 : Inport  LatchInput=off
  Demux1 : Demux  Outputs=b(offset+1:offset+16)
  Matrix Concatenation : simulink/Math Operations/Matrix Concatenation  numInports=16  catMethod=Vertical
  Rectangular QAM Modulator Baseband1 : commdigbbndam2/Rectangular QAM Modulator Baseband  M=2^b(offset+1)  InType=Bit  Enc=Gray  PowType=Average Power  MinDist=2  AvgPow=1  PeakPow=1  Ph=0  numSamp=1
  Rectangular QAM Modulator Baseband10 : commdigbbndam2/Rectangular QAM Modulator Baseband  M=2^b(offset+10)  InType=Bit  Enc=Gray  PowType=Average Power  MinDist=2  AvgPow=1  PeakPow=1  Ph=0  numSamp=1
  Rectangular QAM Modulator Baseband11 : commdigbbndam2/Rectangular QAM Modulator Baseband  M=2^b(offset+11)  InType=Bit  Enc=Gray  PowType=Average Power  MinDist=2  AvgPow=1  PeakPow=1  Ph=0  numSamp=1
  Rectangular QAM Modulator Baseband12 : commdigbbndam2/Rectangular QAM Modulator Baseband  M=2^b(offset+12)  InType=Bit  Enc=Gray  PowType=Average Power  MinDist=2  AvgPow=1  PeakPow=1  Ph=0  numSamp=1
  Rectangular QAM Modulator Baseband13 : commdigbbndam2/Rectangular QAM Modulator Baseband  M=2^b(offset+13)  InType=Bit  Enc=Gray  PowType=Average Power  MinDist=2  AvgPow=1  PeakPow=1  Ph=0  numSamp=1
  Rectangular QAM Modulator Baseband14 : commdigbbndam2/Rectangular QAM Modulator Baseband  M=2^b(offset+14)  InType=Bit  Enc=Gray  PowType=Average Power  MinDist=2  AvgPow=1  PeakPow=1  Ph=0  numSamp=1
  Rectangular QAM Modulator Baseband15 : commdigbbndam2/Rectangular QAM Modulator Baseband  M=2^b(offset+15)  InType=Bit  Enc=Gray  PowType=Average Power  MinDist=2  AvgPow=1  PeakPow=1  Ph=0  numSamp=1
  Rectangular QAM Modulator Baseband16 : commdigbbndam2/Rectangular QAM Modulator Baseband  M=2^b(offset+16)  InType=Bit  Enc=Gray  PowType=Average Power  MinDist=2  AvgPow=1  PeakPow=1  Ph=0  numSamp=1
  Rectangular QAM Modulator Baseband2 : commdigbbndam2/Rectangular QAM Modulator Baseband  M=2^b(offset+2)  InType=Bit  Enc=Gray  PowType=Average Power  MinDist=2  AvgPow=1  PeakPow=1  Ph=0  numSamp=1
  Rectangular QAM Modulator Baseband3 : commdigbbndam2/Rectangular QAM Modulator Baseband  M=2^b(offset+3)  InType=Bit  Enc=Gray  PowType=Average Power  MinDist=2  AvgPow=1  PeakPow=1  Ph=0  numSamp=1
  Rectangular QAM Modulator Baseband4 : commdigbbndam2/Rectangular QAM Modulator Baseband  M=2^b(offset+4)  InType=Bit  Enc=Gray  PowType=Average Power  MinDist=2  AvgPow=1  PeakPow=1  Ph=0  numSamp=1
  Rectangular QAM Modulator Baseband5 : commdigbbndam2/Rectangular QAM Modulator Baseband  M=2^b(offset+5)  InType=Bit  Enc=Gray  PowType=Average Power  MinDist=2  AvgPow=1  PeakPow=1  Ph=0  numSamp=1
  Rectangular QAM Modulator Baseband6 : commdigbbndam2/Rectangular QAM Modulator Baseband  M=2^b(offset+6)  InType=Bit  Enc=Gray  PowType=Average Power  MinDist=2  AvgPow=1  PeakPow=1  Ph=0  numSamp=1
  Rectangular QAM Modulator Baseband7 : commdigbbndam2/Rectangular QAM Modulator Baseband  M=2^b(offset+7)  InType=Bit  Enc=Gray  PowType=Average Power  MinDist=2  AvgPow=1  PeakPow=1  Ph=0  numSamp=1
  Rectangular QAM Modulator Baseband8 : commdigbbndam2/Rectangular QAM Modulator Baseband  M=2^b(offset+8)  InType=Bit  Enc=Gray  PowType=Average Power  MinDist=2  AvgPow=1  PeakPow=1  Ph=0  numSamp=1
  Rectangular QAM Modulator Baseband9 : commdigbbndam2/Rectangular QAM Modulator Baseband  M=2^b(offset+9)  InType=Bit  Enc=Gray  PowType=Average Power  MinDist=2  AvgPow=1  PeakPow=1  Ph=0  numSamp=1
  Out1 : Outport
  wires:
  Rectangular QAM Modulator Baseband16/1 -> Matrix Concatenation/16
  Rectangular QAM Modulator Baseband15/1 -> Matrix Concatenation/15
  Rectangular QAM Modulator Baseband14/1 -> Matrix Concatenation/14
  Rectangular QAM Modulator Baseband13/1 -> Matrix Concatenation/13
  Rectangular QAM Modulator Baseband12/1 -> Matrix Concatenation/12
  Rectangular QAM Modulator Baseband11/1 -> Matrix Concatenation/11
  Rectangular QAM Modulator Baseband10/1 -> Matrix Concatenation/10
  Rectangular QAM Modulator Baseband9/1 -> Matrix Concatenation/9
  Rectangular QAM Modulator Baseband8/1 -> Matrix Concatenation/8
  Rectangular QAM Modulator Baseband7/1 -> Matrix Concatenation/7
  Rectangular QAM Modulator Baseband6/1 -> Matrix Concatenation/6
  Rectangular QAM Modulator Baseband5/1 -> Matrix Concatenation/5
  Rectangular QAM Modulator Baseband4/1 -> Matrix Concatenation/4
  Rectangular QAM Modulator Baseband3/1 -> Matrix Concatenation/3
  Rectangular QAM Modulator Baseband2/1 -> Matrix Concatenation/2
  Demux1/16 -> Rectangular QAM Modulator Baseband16/1
  Demux1/15 -> Rectangular QAM Modulator Baseband15/1
  Demux1/14 -> Rectangular QAM Modulator Baseband14/1
  Demux1/13 -> Rectangular QAM Modulator Baseband13/1
  Demux1/12 -> Rectangular QAM Modulator Baseband12/1
  Demux1/11 -> Rectangular QAM Modulator Baseband11/1
  Demux1/10 -> Rectangular QAM Modulator Baseband10/1
  Demux1/9 -> Rectangular QAM Modulator Baseband9/1
  Demux1/8 -> Rectangular QAM Modulator Baseband8/1
  Demux1/7 -> Rectangular QAM Modulator Baseband7/1
  Demux1/6 -> Rectangular QAM Modulator Baseband6/1
  Demux1/5 -> Rectangular QAM Modulator Baseband5/1
  Demux1/4 -> Rectangular QAM Modulator Baseband4/1
  Demux1/3 -> Rectangular QAM Modulator Baseband3/1
  Matrix Concatenation/1 -> Out1/1
  In1/1 -> Demux1/1
  Demux1/2 -> Rectangular QAM Modulator Baseband2/1
  Demux1/1 -> Rectangular QAM Modulator Baseband1/1
  Rectangular QAM Modulator Baseband1/1 -> Matrix Concatenation/1
